simulink model "project_training_data"  (R2023b)
settings: Solver=FixedStepAuto  StartTime=0.0  StopTime=75  FixedStep=0.025  RelTol=1e-3
model workspace (MAT data in the model file):
  A = Simulink.Parameter
  A.Value = [1  0.025  0  0  0  0; 0  1  0  0  0  0; 0  0  1  0.025  0  0; 0  0  0  1  0  0; 0  0  0  0  1  0.025; 0  0  0  0  0  1]
  A.DataType = 'auto'
  A.Complexity = 'real'
  A.Dimensions = [6 6]
  Aag = Simulink.Parameter
  Aag.Value = [1  0.025  0  0  0  0; 0  1  0  0  0  0; 0  0  1  0.025  0  0; 0  0  0  1  0  0; 0  0  0  0  1  0.025; 0  0  0  0  0  1]
  Aag.DataType = 'auto'
  Aag.Complexity = 'real'
  Aag.Dimensions = [6 6]
  B = Simulink.Parameter
  B.Value = [-0.003065625  0  0; -0.24525  0  0; 0  0.003065625  0; 0  0.24525  0; 0  0  0.0003125; 0  0  0.025]
  B.DataType = 'auto'
  B.Complexity = 'real'
  B.Dimensions = [6 3]
  Bag = Simulink.Parameter
  Bag.Value = [0.0416666666667  0  0; 3.33333333333  0  0; 0  0.0416666666667  0; 0  3.33333333333  0; 0  0  0.0240384615385; 0  0  1.92307692308]
  Bag.DataType = 'auto'
  Bag.Complexity = 'real'
  Bag.Dimensions = [6 3]
  C = Simulink.Parameter
  C.Value = [1  0  0  0  0  0; 0  0  1  0  0  0; 0  0  0  0  1  0]
  C.DataType = 'auto'
  C.Complexity = 'real'
  C.Dimensions = [3 6]
  Cag = Simulink.Parameter
  Cag.Value = [1  0  0  0  0  0; 0  0  1  0  0  0; 0  0  0  0  1  0]
  Cag.DataType = 'auto'
  Cag.Complexity = 'real'
  Cag.Dimensions = [3 6]
  uang = [0 0 0 0 0 0 5.50670620214e-14 5.44009282066e-14 0 -3.99756362155e-05 -2.83106871279e-14 0 ... (9003 elements, 3x3001)]
  upos = [0 0 0 5.62466739851e-14 5.62327961973e-14 0 -2.39975660277e-05 4.94743135349e-14 0 -9.31686537426e-05 7.62168106405e-14 0 ... (9003 elements, 3x3001)]
libraries: aerolibanimutils x1
(part 1 of 2)
settings Model: Creator=Lingf  LastModifiedBy=deandre
settings SolverCC: AlgebraicLoopSolver=TrustRegion
settings DataIOCC: ReturnWorkspaceOutputs=off
settings DebuggingCC: UnconnectedInputMsg=warning  UnconnectedOutputMsg=warning  UnconnectedLineMsg=warning
settings ModelReferenceCC: EnableRefExpFcnMdlSchedulingChecks=on
settings RTWCC: DLArmComputeVersion=19.05

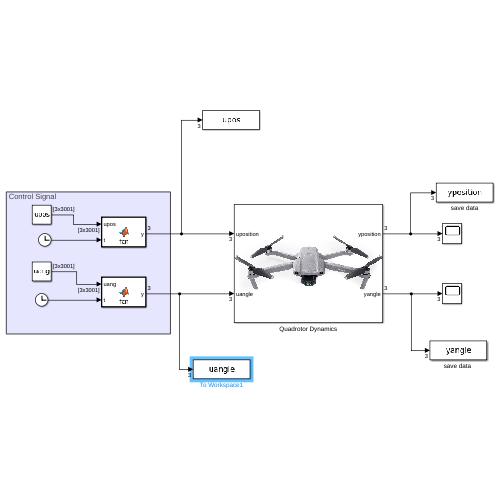
[thumbnail: Simulink's stored preview of the top-level diagram]
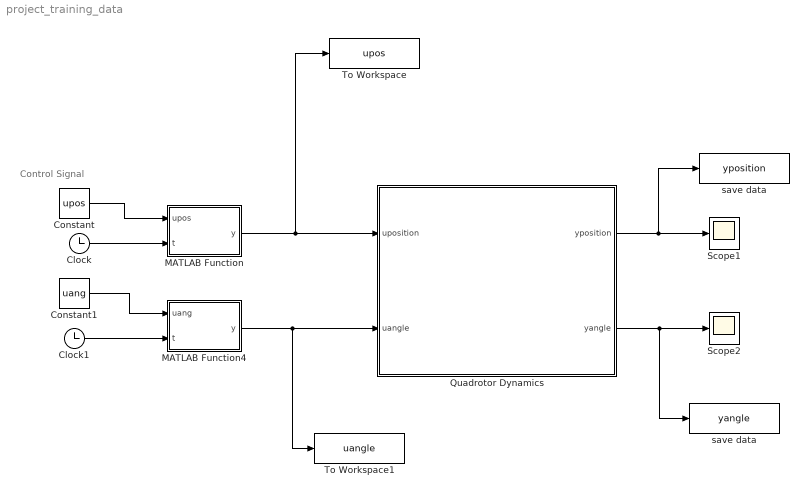
== system project_training_data ==
  note: Control Signal
  Clock : Clock
  Clock1 : Clock
  Constant : Constant  Value=upos
  Constant1 : Constant  Value=uang
  MATLAB Function : MATLAB Function  TreatAsAtomicUnit=on
  MATLAB Function4 : MATLAB Function  TreatAsAtomicUnit=on
  Quadrotor Dynamics : Subsystem
      mask Display: image('$imagefile'); % Use "Edit Image" on toolstrip to change.
  Scope1 : Scope
  Scope2 : Scope
  To Workspace : ToWorkspace  VariableName=upos  SampleTime=-1
      settings: Save2DSignal=2-D array (concatenate along first dimension)
  To Workspace1 : ToWorkspace  VariableName=uangle  SampleTime=-1
      settings: Save2DSignal=2-D array (concatenate along first dimension)
  save data : ToWorkspace  VariableName=yposition  SampleTime=-1
      settings: Save2DSignal=2-D array (concatenate along first dimension)
  "save data " : ToWorkspace  VariableName=yangle  SampleTime=-1
      settings: Save2DSignal=2-D array (concatenate along first dimension)
  wires:
  Clock/1 -> MATLAB Function/2(t)
  Clock1/1 -> MATLAB Function4/2(t)
  Constant/1 -> MATLAB Function/1(upos)
  Constant1/1 -> MATLAB Function4/1(uang)
  Quadrotor Dynamics/1(yposition) -> save data/1, Scope1/1
  Quadrotor Dynamics/2(yangle) -> "save data "/1, Scope2/1
  MATLAB Function/1(y) -> To Workspace/1, Quadrotor Dynamics/1(uposition)
  MATLAB Function4/1(y) -> To Workspace1/1, Quadrotor Dynamics/2(uangle)
